simulink model "SaturationUsingMiniMax"  (R2013a)
settings: Solver=ode45  StartTime=0.0  StopTime=10.0  RelTol=1e-3
settings Model: Creator=ajdin  LastModifiedBy=ajdin

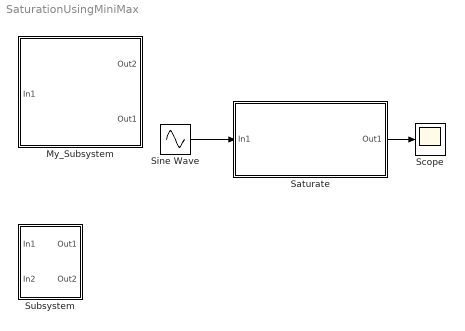
== system SaturationUsingMiniMax ==
  My_Subsystem : Subsystem  mask{GAIN=87}
      mask init:
      | if(GAIN>5)
      |     Thresh=0.1;
      |     
      | else 
      |     Thresh=0.01;
      |     
      | end
      mask Display:
      | disp('my|sys');
      | color('blue');
      | 
      | port_label('output', 1, 'out');
      | port_label('output', 2, 'Thresh');
      | port_label('input', 1, 'signal');
  Saturate : Subsystem
      mask Display:
      | disp('Saturate');
      | color('blue');
      | port_label('output', 1, 'output');
      | port_label('input', 1, 'signal');
  Scope : Scope
  Sine Wave : Sin  Amplitude=5  SampleTime=0
  Subsystem : Subsystem
      mask Display:
      | color('blue');
      | 
      | port_label('output', 1, 'add');
      | port_label('output', 2, '');
      | port_label('input', 1, 'in1');
      | port_label('input', 2, 'in2');
  wires:
  Sine Wave/1 -> Saturate/1(In1)
  Saturate/1(Out1) -> Scope/1

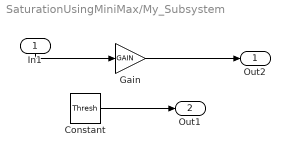
== system SaturationUsingMiniMax/My_Subsystem ==
  In1 : Inport
  Constant : Constant  Value=Thresh
  Gain : Gain  Gain=GAIN
  Out2 : Outport
  Out1 : Outport  Port=2
  wires:
  In1/1 -> Gain/1
  Gain/1 -> Out2/1
  Constant/1 -> Out1/1

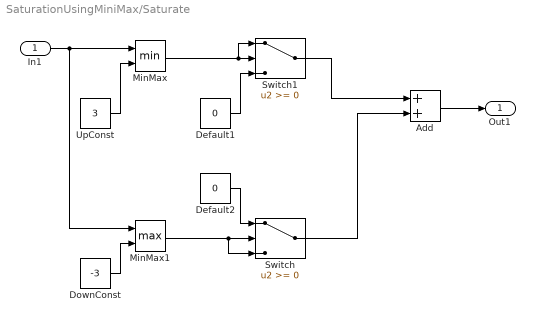
== system SaturationUsingMiniMax/Saturate ==
  In1 : Inport
  Add : Sum
  Default1 : Constant  Value=0
  Default2 : Constant  Value=0
  DownConst : Constant  Value=-3
  MinMax : MinMax  Inputs=2
  MinMax1 : MinMax  Function=max  Inputs=2
  Switch : Switch
  Switch1 : Switch
  UpConst : Constant  Value=3
  Out1 : Outport
  wires:
  Switch/1 -> Add/2
  Switch1/1 -> Add/1
  Add/1 -> Out1/1
  In1/1 -> MinMax1/1, MinMax/1
  UpConst/1 -> MinMax/2
  DownConst/1 -> MinMax1/2
  MinMax/1 -> Switch1/1, Switch1/2
  Default1/1 -> Switch1/3
  MinMax1/1 -> Switch/2, Switch/3
  Default2/1 -> Switch/1

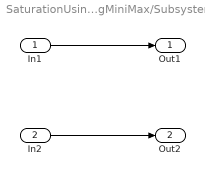
== system SaturationUsingMiniMax/Subsystem ==
  In1 : Inport
  In2 : Inport  Port=2
  Out1 : Outport
  Out2 : Outport  Port=2
  wires:
  In1/1 -> Out1/1
  In2/1 -> Out2/1
